simulink model "chap1_3"  (R2023b)
settings: Solver=ode45  StartTime=0.0  StopTime=10.0  RelTol=1e-3
settings Model: Creator=CorgiQvm  LastModifiedBy=CorgiQvm
settings DataIOCC: ReturnWorkspaceOutputs=off

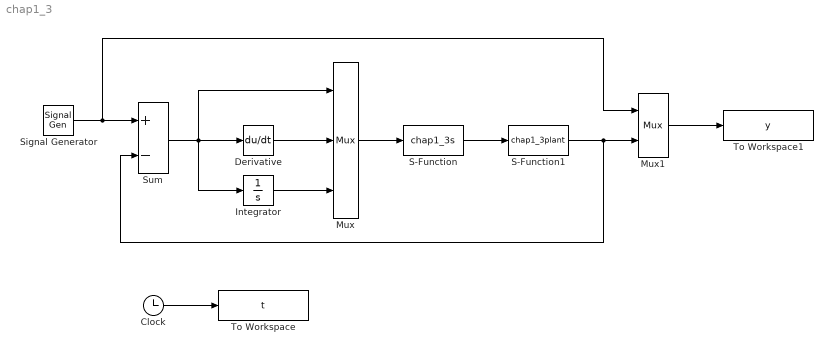
== system chap1_3 ==
  Clock : Clock
  Derivative : Derivative
  Integrator : Integrator
  Mux : Mux  Inputs=3
  Mux1 : Mux  Inputs=2
  S-Function : S-Function  FunctionName=chap1_3s  SFunctionDeploymentMode=off  EnableBusSupport=off
  S-Function1 : S-Function  FunctionName=chap1_3plant  SFunctionDeploymentMode=off  EnableBusSupport=off
  Signal Generator : SignalGenerator  Frequency=0.2
  Sum : Sum  Inputs=+-  InputSameDT=on  SaturateOnIntegerOverflow=on  OutDataTypeStr=Inherit: Same as first input
  To Workspace : ToWorkspace  VariableName=t  SampleTime=-1
  To Workspace1 : ToWorkspace  VariableName=y  SampleTime=-1
  wires:
  Signal Generator/1 -> Mux1/1, Sum/1
  Sum/1 -> Mux/1, Integrator/1, Derivative/1
  Derivative/1 -> Mux/2
  Mux/1 -> S-Function/1
  S-Function/1 -> S-Function1/1
  S-Function1/1 -> Sum/2, Mux1/2
  Mux1/1 -> To Workspace1/1
  Integrator/1 -> Mux/3
  Clock/1 -> To Workspace/1
